simulink model "merge_test_tmp"  (Simulink 8.3)
settings: Solver=VariableStepDiscrete  StartTime=0.0  StopTime=0  MaxStep=1  RelTol=1e-3
settings Model: Creator=arnaud  LastModifiedBy=hbourbou
settings DataIOCC: ExternalInput=xin  SaveFormat=Structure
settings OptimizationCC: ExpressionDepthLimit=2147483647
settings DebuggingCC: FcnCallInpInsideContextMsg=EnableAllAsWarning  FrameProcessingCompatibilityMsg=error

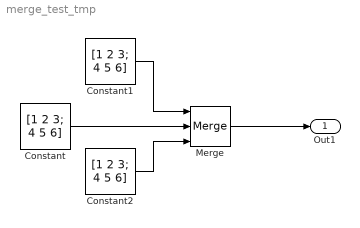
== system merge_test_tmp ==
  Constant : Constant  Value=[1 2 3; 4 5 6]
  Constant1 : Constant  Value=[1 2 3; 4 5 6]
  Constant2 : Constant  Value=[1 2 3; 4 5 6]
  Merge : Merge  Inputs=3
  Out1 : Outport
  wires:
  Merge/1 -> Out1/1
  Constant1/1 -> Merge/1
  Constant/1 -> Merge/2
  Constant2/1 -> Merge/3
